simulink model "torqueBalancingPHRIStandup"  (Simulink 9.1)
settings: Solver=FixedStepDiscrete  StartTime=0.0  StopTime="Config.SIMULATION_TIME "  FixedStep=Config.Ts  RelTol=1e-3  EnableMultiTasking=on
StopFcn:
  | cd(fileparts(which(bdroot)));
  | stopTorqueBalancingPHRIStandup;
undefined symbols (not defined in the file or in its folder): ASSISTANT_DOF_FOR_SIMULINK, bVectorConstraintsFeet, bVectorConstraintsLegs, Config, ConstraintsMatrixFeet, ConstraintsMatrixLegs, Gain, Reg, ROBOT_DOF, ROBOT_DOF_FOR_SIMULINK, Sat, Sm
libraries: WBToolboxLibrary x154, simulink x4
(part 2 of 4)

== system torqueBalancingPHRIStandup/Robot system/Dynamics and Kinematics/Dynamics ==
  w_H_b : Inport
  qj : Inport  Port=2
  nu : Inport  Port=3
  Add motors reflected inertias : Subsystem
  Centroidal Momentum : WBToolboxLibrary/wholeBodyModel/Dynamics/Centroidal Momentum
      settings: SourceProductName=Whole Body Toolbox
  "CoM6D ->  CoMXYZ1" : Selector  InputPortWidth=6+ROBOT_DOF  IndexOptions=Index vector (dialog)  Indices=[7:6+ROBOT_DOF]  OutputSizes=1
  "CoM6D ->  CoMXYZ2" : Selector  InputPortWidth=6+ROBOT_DOF  IndexOptions=Index vector (dialog)  Indices=[1 2 3 4 5 6]  OutputSizes=1
  Get Bias Forces : WBToolboxLibrary/wholeBodyModel/Dynamics/Get Bias Forces
      settings: SourceProductName=Whole Body Toolbox
  Mass Matrix : WBToolboxLibrary/wholeBodyModel/Dynamics/Mass Matrix
      settings: SourceProductName=Whole Body Toolbox
  M(q) : Outport
  biasTorques : Outport  Port=2
  L(q,dq) : Outport  Port=3
  wires:
  Mass Matrix/1 -> Add motors reflected inertias/1(M)
  Centroidal Momentum/1 -> L(q,dq)/1
  Get Bias Forces/1 -> biasTorques/1
  w_H_b/1 -> Centroidal Momentum/1, Get Bias Forces/1, Mass Matrix/1
  qj/1 -> Centroidal Momentum/2, Get Bias Forces/2, Mass Matrix/2
  "CoM6D ->  CoMXYZ2"/1 -> Centroidal Momentum/3, Get Bias Forces/3
  "CoM6D ->  CoMXYZ1"/1 -> Centroidal Momentum/4, Get Bias Forces/4
  nu/1 -> "CoM6D ->  CoMXYZ1"/1, "CoM6D ->  CoMXYZ2"/1
  Add motors reflected inertias/1(M_with_motor_inertia) -> M(q)/1

== system torqueBalancingPHRIStandup/Robot system/Dynamics and Kinematics/Kinematics ==
  nu : Inport
  qj : Inport  Port=2
  w_H_b : Inport  Port=3
  "state " : Inport  Port=4
  Arm Contacts Kinematics : Subsystem
  "CoM6D ->  CoMXYZ3" : Selector  InputPortWidth=6+ROBOT_DOF  IndexOptions=Index vector (dialog)  Indices=[7:6+ROBOT_DOF]  OutputSizes=1
  "CoM6D ->  CoMXYZ4" : Selector  InputPortWidth=6+ROBOT_DOF  IndexOptions=Index vector (dialog)  Indices=[1 2 3 4 5 6]  OutputSizes=1
  Constant : Constant  Value=Config.iCubStandUp
  Contacts kinematics : Subsystem
  Jacobian com : WBToolboxLibrary/wholeBodyModel/Jacobians/Jacobian  frameName=Frames.COM
      settings: SourceProductName=Whole Body Toolbox
  Legs in Contact : MATLAB Function  TreatAsAtomicUnit=on
  xCom : Subsystem
  w_H_l_contact : Outport
  w_H_r_contact : Outport  Port=2
  J_l_contact : Outport  Port=3
  J_r_contact : Outport  Port=4
  J_CoM : Outport  Port=5
  xCoM : Outport  Port=6
  JDot_nu_l_contact : Outport  Port=7
  JDot_nu_r_contact : Outport  Port=8
  legsInContact : Outport  Port=9
  w_H_lArmContact : Outport  Port=10
  w_H_rArmContact : Outport  Port=11
  JLArm : Outport  Port=12
  JRArm : Outport  Port=13
  JDot_nu_lArm_contact : Outport  Port=14
  JDot_nu_rArm_contact : Outport  Port=15
  wires:
  nu/1 -> "CoM6D ->  CoMXYZ3"/1, "CoM6D ->  CoMXYZ4"/1
  w_H_b/1 -> Arm Contacts Kinematics/1(w_H_b1), Contacts kinematics/1(w_H_b), xCom/1(w_H_b), Jacobian com/1
  qj/1 -> Jacobian com/2, Arm Contacts Kinematics/2(qj1), Contacts kinematics/2(qj), xCom/2(qj)
  Jacobian com/1 -> J_CoM/1
  xCom/1(xCoM) -> xCoM/1
  "state "/1 -> Legs in Contact/2(state)
  Constant/1 -> Legs in Contact/1(icubStandup)
  "CoM6D ->  CoMXYZ3"/1 -> Arm Contacts Kinematics/4(dqj), Contacts kinematics/4(dqj)
  "CoM6D ->  CoMXYZ4"/1 -> Arm Contacts Kinematics/3(nu_b), Contacts kinematics/3(nu_b)
  Legs in Contact/1(legsInContact) -> Contacts kinematics/5(legsInContact), legsInContact/1
  Contacts kinematics/1(w_H_lContact) -> w_H_l_contact/1
  Contacts kinematics/2(w_H_rContact) -> w_H_r_contact/1
  Contacts kinematics/5(dJLnu) -> JDot_nu_l_contact/1
  Contacts kinematics/6(dJRnu) -> JDot_nu_r_contact/1
  Contacts kinematics/3(JL) -> J_l_contact/1
  Contacts kinematics/4(JR) -> J_r_contact/1
  Arm Contacts Kinematics/4(JRArm) -> JRArm/1
  Arm Contacts Kinematics/5(dJLArmnu) -> JDot_nu_lArm_contact/1
  Arm Contacts Kinematics/3(JLArm) -> JLArm/1
  Arm Contacts Kinematics/1(w_H_lArmContact) -> w_H_lArmContact/1
  Arm Contacts Kinematics/6(dJRArmnu) -> JDot_nu_rArm_contact/1
  Arm Contacts Kinematics/2(w_H_rArmContact) -> w_H_rArmContact/1

== system torqueBalancingPHRIStandup/Robot system/Robot State and References/Centroidal Momentum Matrix  ==
  w_H_b : Inport
  jointPos : Inport  Port=2
  CMM_LArm : Subsystem
  CMM_LLeg : Subsystem
  CMM_RArm : Subsystem
  CMM_RLeg : Subsystem
  CMM_base : Subsystem
  CMM_torso : Subsystem
  Matrix Concatenate6 : Concatenate  NumInputs=6  Mode=Multidimensional array  ConcatenateDimension=2
  CMM : Outport
  wires:
  Matrix Concatenate6/1 -> CMM/1
  CMM_base/1(CMM_base) -> Matrix Concatenate6/1
  CMM_torso/1(CMM_torso) -> Matrix Concatenate6/2
  CMM_LArm/1(CMM_LArm) -> Matrix Concatenate6/3
  jointPos/1 -> CMM_LArm/2(jointPos), CMM_RLeg/2(jointPos), CMM_LLeg/2(jointPos), CMM_RArm/2(jointPos), CMM_torso/2(jointPos), CMM_base/2(jointPos)
  w_H_b/1 -> CMM_LArm/1(w_H_b), CMM_RLeg/1(w_H_b), CMM_LLeg/1(w_H_b), CMM_RArm/1(w_H_b), CMM_torso/1(w_H_b), CMM_base/1(w_H_b)
  CMM_RArm/1(CMM_RArm) -> Matrix Concatenate6/4
  CMM_LLeg/1(CMM_LLeg) -> Matrix Concatenate6/5
  CMM_RLeg/1(CMM_RLeg) -> Matrix Concatenate6/6

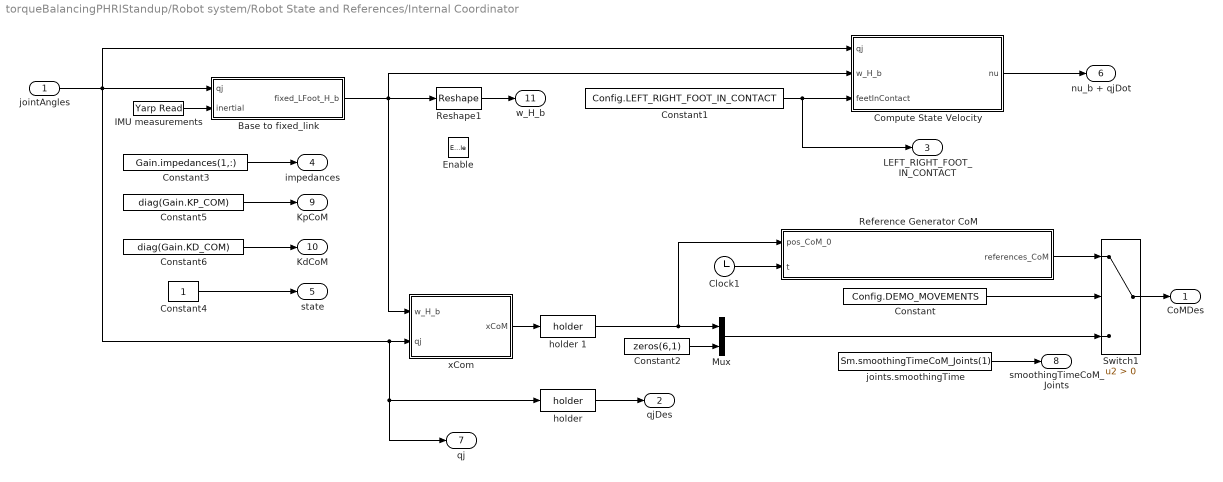
== system torqueBalancingPHRIStandup/Robot system/Robot State and References/Internal Coordinator ==
  jointAngles : Inport
  Enable : EnablePort
  Base to fixed_link : Subsystem
  Clock1 : Clock
  Compute State Velocity : Subsystem
  Constant : Constant  Value=Config.DEMO_MOVEMENTS
  Constant1 : Constant  Value=Config.LEFT_RIGHT_FOOT_IN_CONTACT
  Constant2 : Constant  Value=zeros(6,1)
  Constant3 : Constant  Value=Gain.impedances(1,:)
  Constant4 : Constant
  Constant5 : Constant  Value=diag(Gain.KP_COM)
  Constant6 : Constant  Value=diag(Gain.KD_COM)
  IMU measurements : WBToolboxLibrary/Utilities/Yarp Read  portName=Ports.IMU  signalSize=12  timeout=0.5  blocking=off  timestamp=off  autoconnect=on  errorOnConnection=on
      settings: SourceProductName=Whole Body Toolbox
  Mux : Mux  Inputs=2
  Reference Generator CoM : MATLAB Function  TreatAsAtomicUnit=on
  Reshape1 : Reshape  OutputDimensions=[4;4]
  Switch1 : Switch  Criteria=u2 > Threshold
  "holder " : WBToolboxLibrary/Utilities/holder 
      settings: SourceProductName=Whole Body Toolbox
  holder 1 : WBToolboxLibrary/Utilities/holder 
      settings: SourceProductName=Whole Body Toolbox
  joints.smoothingTime : Constant  Value=Sm.smoothingTimeCoM_Joints(1)
  xCom : Subsystem
  CoMDes : Outport
  qjDes : Outport  Port=2
  LEFT_RIGHT_FOOT_IN_CONTACT : Outport  Port=3
  impedances : Outport  Port=4
  state : Outport  Port=5
  nu_b + qjDot : Outport  Port=6
  qj : Outport  Port=7
  smoothingTimeCoM_Joints : Outport  Port=8
  KpCoM : Outport  Port=9
  KdCoM : Outport  Port=10
  w_H_b : Outport  Port=11
  wires:
  Constant/1 -> Switch1/2
  "holder "/1 -> qjDes/1
  Switch1/1 -> CoMDes/1
  Mux/1 -> Switch1/3
  Constant2/1 -> Mux/2
  Constant3/1 -> impedances/1
  Constant4/1 -> state/1
  Compute State Velocity/1(nu) -> nu_b + qjDot/1
  holder 1/1 -> Reference Generator CoM/1(pos_CoM_0), Mux/1
  Base to fixed_link/1(fixed_LFoot_H_b) -> Compute State Velocity/2(w_H_b), xCom/1(w_H_b), Reshape1/1
  xCom/1(xCoM) -> holder 1/1
  joints.smoothingTime/1 -> smoothingTimeCoM_Joints/1
  jointAngles/1 -> Compute State Velocity/1(qj), Base to fixed_link/1(qj), qj/1, "holder "/1, xCom/2(qj)
  Constant5/1 -> KpCoM/1
  Constant6/1 -> KdCoM/1
  Reshape1/1 -> w_H_b/1
  Constant1/1 -> Compute State Velocity/3("feetInContact "), LEFT_RIGHT_FOOT_IN_CONTACT/1
  IMU measurements/1 -> Base to fixed_link/2(inertial)
  Clock1/1 -> Reference Generator CoM/2(t)
  Reference Generator CoM/1(references_CoM) -> Switch1/1

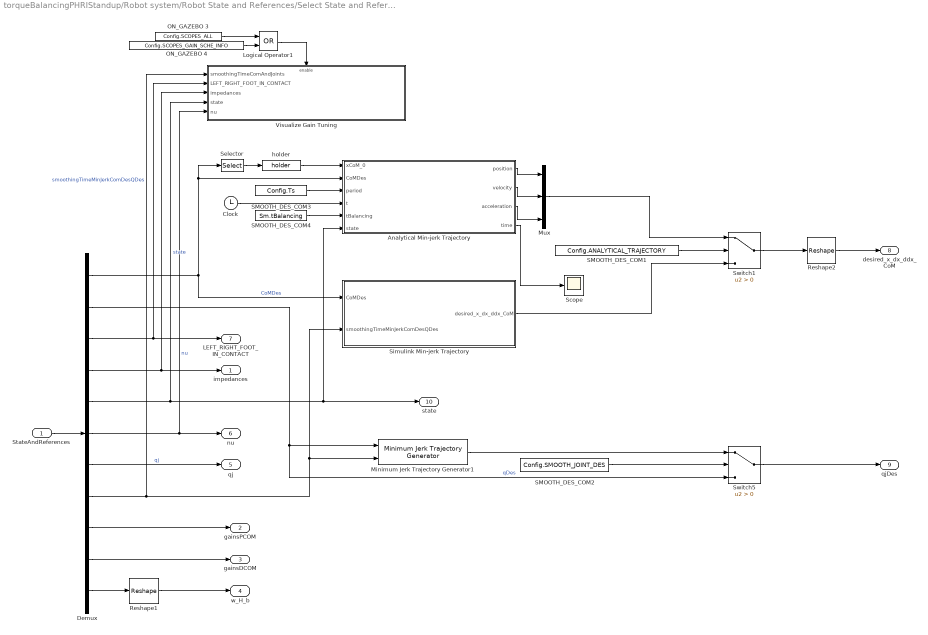
== system torqueBalancingPHRIStandup/Robot system/Robot State and References/Select State and References ==
  StateAndReferences : Inport
  Analytical Min-jerk Trajectory : MATLAB Function  TreatAsAtomicUnit=on
  Clock : Clock
  Demux : Demux  Outputs=[9,ROBOT_DOF,2,ROBOT_DOF,1,ROBOT_DOF+6,ROBOT_DOF,1,3,3,16]
  Logical Operator1 : Logic  Operator=OR  AllPortsSameDT=off  OutDataTypeStr=boolean
  Minimum Jerk Trajectory Generator1 : WBToolboxLibrary/Utilities/Minimum Jerk Trajectory Generator  externalSettlingTime=on  settlingTime=1  sampleTime=Config.Ts  resetOnSettlingTime=off  firstDerivatives=off  secondDerivatives=off  explicitInitialValue=off
      settings: SourceProductName=Whole Body Toolbox
  Mux : Mux  Inputs=3
  ON_GAZEBO 3 : Constant  Value=Config.SCOPES_ALL
  ON_GAZEBO 4 : Constant  Value=Config.SCOPES_GAIN_SCHE_INFO
  Reshape1 : Reshape  OutputDimensionality=Customize  OutputDimensions=[4;4]
  Reshape2 : Reshape  OutputDimensionality=Customize  OutputDimensions=[3,3]
  SMOOTH_DES_COM1 : Constant  Value=Config.ANALYTICAL_TRAJECTORY
  SMOOTH_DES_COM2 : Constant  Value=Config.SMOOTH_JOINT_DES
  SMOOTH_DES_COM3 : Constant  Value=Config.Ts
  SMOOTH_DES_COM4 : Constant  Value=Sm.tBalancing
  Scope : Scope
  Selector : Selector  InputPortWidth=9  IndexOptions=Index vector (dialog)  Indices=[1 2 3]  OutputSizes=1
  "Simulink Min-jerk Trajectory " : Subsystem
  Switch1 : Switch  Criteria=u2 > Threshold
  Switch5 : Switch  Criteria=u2 > Threshold
  "Visualize Gain Tuning  " : Subsystem
  "holder " : WBToolboxLibrary/Utilities/holder 
      settings: SourceProductName=Whole Body Toolbox
  impedances : Outport
  gainsPCOM : Outport  Port=2
  gainsDCOM : Outport  Port=3
  w_H_b : Outport  Port=4
  qj : Outport  Port=5
  nu : Outport  Port=6
  LEFT_RIGHT_FOOT_IN_CONTACT : Outport  Port=7
  desired_x_dx_ddx_CoM : Outport  Port=8
  qjDes : Outport  Port=9
  state : Outport  Port=10
  wires:
  SMOOTH_DES_COM2/1 -> Switch5/2
  Switch5/1 -> qjDes/1
  Demux/7 -> qj/1  "qj"
  Demux/11 -> Reshape1/1
  Demux/5 -> "Visualize Gain Tuning  "/4(state), Analytical Min-jerk Trajectory/6(state), state/1  "state"
  Demux/8 -> Minimum Jerk Trajectory Generator1/2, "Simulink Min-jerk Trajectory "/2(smoothingTimeMinJerkComDesQDes), "Visualize Gain Tuning  "/1(smoothingTimeComAndJoints)  "smoothingTimeMinJerkComDesQDes"
  Demux/2 -> Minimum Jerk Trajectory Generator1/1, Switch5/3  "qDes"
  Minimum Jerk Trajectory Generator1/1 -> Switch5/1
  Demux/6 -> "Visualize Gain Tuning  "/5(nu), nu/1  "nu"
  StateAndReferences/1 -> Demux/1
  Demux/4 -> "Visualize Gain Tuning  "/3(impedances), impedances/1
  Demux/3 -> "Visualize Gain Tuning  "/2(LEFT_RIGHT_FOOT_IN_CONTACT), LEFT_RIGHT_FOOT_IN_CONTACT/1
  Demux/9 -> gainsPCOM/1
  Demux/10 -> gainsDCOM/1
  Reshape1/1 -> w_H_b/1
  ON_GAZEBO 4/1 -> Logical Operator1/2
  ON_GAZEBO 3/1 -> Logical Operator1/1
  Logical Operator1/1 -> "Visualize Gain Tuning  "/Enable
  Demux/1 -> "Simulink Min-jerk Trajectory "/1(CoMDes), Selector/1, Analytical Min-jerk Trajectory/2(CoMDes)  "CoMDes"
  SMOOTH_DES_COM1/1 -> Switch1/2
  Switch1/1 -> Reshape2/1
  "Simulink Min-jerk Trajectory "/1(desired_x_dx_ddx_CoM) -> Switch1/3
  SMOOTH_DES_COM3/1 -> Analytical Min-jerk Trajectory/3(period)
  Clock/1 -> Analytical Min-jerk Trajectory/4(t)
  SMOOTH_DES_COM4/1 -> Analytical Min-jerk Trajectory/5(tBalancing)
  Reshape2/1 -> desired_x_dx_ddx_CoM/1
  Selector/1 -> "holder "/1
  "holder "/1 -> Analytical Min-jerk Trajectory/1(xCoM_0)
  Analytical Min-jerk Trajectory/1(position) -> Mux/1
  Analytical Min-jerk Trajectory/2(velocity) -> Mux/2
  Analytical Min-jerk Trajectory/3(acceleration) -> Mux/3
  Mux/1 -> Switch1/1
  Analytical Min-jerk Trajectory/4(time) -> Scope/1

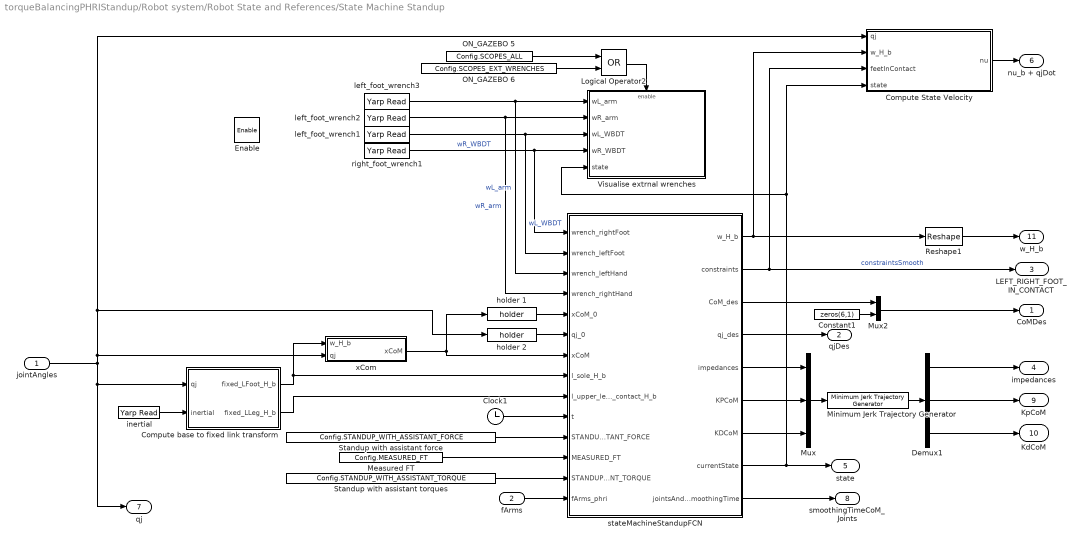
== system torqueBalancingPHRIStandup/Robot system/Robot State and References/State Machine Standup ==
  jointAngles : Inport
  fArms : Inport  Port=2
  Enable : EnablePort
  Clock1 : Clock
  Compute State Velocity : Subsystem
  Compute base to fixed link transform : Subsystem
  Constant1 : Constant  Value=zeros(6,1)
  Demux1 : Demux  Outputs=[ROBOT_DOF,3,3]
  Logical Operator2 : Logic  Operator=OR  AllPortsSameDT=off  OutDataTypeStr=boolean
  Measured FT : Constant  Value=Config.MEASURED_FT
  Minimum Jerk Trajectory Generator : WBToolboxLibrary/Utilities/Minimum Jerk Trajectory Generator  externalSettlingTime=off  settlingTime=Gain.SmoothingTimeGainScheduling  sampleTime=Config.Ts  resetOnSettlingTime=off  firstDerivatives=off  secondDerivatives=off  explicitInitialValue=off
      settings: SourceProductName=Whole Body Toolbox
  Mux : Mux  Inputs=3
  Mux2 : Mux  Inputs=2
  ON_GAZEBO 5 : Constant  Value=Config.SCOPES_ALL
  ON_GAZEBO 6 : Constant  Value=Config.SCOPES_EXT_WRENCHES
  Reshape1 : Reshape  OutputDimensions=[4;4]
  Standup with assistant force : Constant  Value=Config.STANDUP_WITH_ASSISTANT_FORCE
  Standup with assistant torques : Constant  Value=Config.STANDUP_WITH_ASSISTANT_TORQUE
  Visualise extrnal wrenches : Subsystem
  holder 1 : WBToolboxLibrary/Utilities/holder 
      settings: SourceProductName=Whole Body Toolbox
  holder 2 : WBToolboxLibrary/Utilities/holder 
      settings: SourceProductName=Whole Body Toolbox
  inertial : WBToolboxLibrary/Utilities/Yarp Read  portName=Ports.IMU  signalSize=12  timeout=0.5  blocking=off  timestamp=off  autoconnect=on  errorOnConnection=off
      settings: SourceProductName=Whole Body Toolbox
  left_foot_wrench1 : WBToolboxLibrary/Utilities/Yarp Read  portName=Ports.WBD_LEFTLEG_EE  signalSize=6  timeout=0.5  blocking=off  timestamp=off  autoconnect=on  errorOnConnection=on
      settings: SourceProductName=Whole Body Toolbox
  left_foot_wrench2 : WBToolboxLibrary/Utilities/Yarp Read  portName=Ports.RIGHT_ARM  signalSize=6  timeout=0.5  blocking=off  timestamp=off  autoconnect=on  errorOnConnection=on
      settings: SourceProductName=Whole Body Toolbox
  left_foot_wrench3 : WBToolboxLibrary/Utilities/Yarp Read  portName=Ports.LEFT_ARM  signalSize=6  timeout=0.5  blocking=off  timestamp=off  autoconnect=on  errorOnConnection=on
      settings: SourceProductName=Whole Body Toolbox
  right_foot_wrench1 : WBToolboxLibrary/Utilities/Yarp Read  portName=Ports.WBD_RIGHTLEG_EE  signalSize=6  timeout=0.5  blocking=off  timestamp=off  autoconnect=on  errorOnConnection=on
      settings: SourceProductName=Whole Body Toolbox
  stateMachineStandupFCN : MATLAB Function  TreatAsAtomicUnit=on
  xCom : Subsystem
  CoMDes : Outport
  qjDes : Outport  Port=2
  LEFT_RIGHT_FOOT_IN_CONTACT : Outport  Port=3
  impedances : Outport  Port=4
  state : Outport  Port=5
  nu_b + qjDot : Outport  Port=6
  qj : Outport  Port=7
  smoothingTimeCoM_Joints : Outport  Port=8
  KpCoM : Outport  Port=9
  KdCoM : Outport  Port=10
  w_H_b : Outport  Port=11
  wires:
  xCom/1(xCoM) -> holder 1/1, stateMachineStandupFCN/7(xCoM)
  stateMachineStandupFCN/4(qj_des) -> qjDes/1
  stateMachineStandupFCN/3(CoM_des) -> Mux2/1
  Mux2/1 -> CoMDes/1
  Constant1/1 -> Mux2/2
  stateMachineStandupFCN/8(currentState) -> Visualise extrnal wrenches/5(state), Compute State Velocity/4("state "), state/1
  stateMachineStandupFCN/2(constraints) -> Compute State Velocity/3("feetInContact "), LEFT_RIGHT_FOOT_IN_CONTACT/1  "constraintsSmooth"
  stateMachineStandupFCN/1(w_H_b) -> Compute State Velocity/2(w_H_b), Reshape1/1
  Compute State Velocity/1(nu) -> nu_b + qjDot/1
  stateMachineStandupFCN/9(jointsAndCoMSmoothingTime) -> smoothingTimeCoM_Joints/1
  stateMachineStandupFCN/6(KPCoM) -> Mux/2
  Demux1/3 -> KdCoM/1
  stateMachineStandupFCN/7(KDCoM) -> Mux/3
  stateMachineStandupFCN/5(impedances) -> Mux/1
  Mux/1 -> Minimum Jerk Trajectory Generator/1
  Minimum Jerk Trajectory Generator/1 -> Demux1/1
  Demux1/1 -> impedances/1
  Demux1/2 -> KpCoM/1
  jointAngles/1 -> Compute State Velocity/1(qj), holder 2/1, xCom/2(qj), qj/1, Compute base to fixed link transform/1(qj)
  Compute base to fixed link transform/1(fixed_LFoot_H_b) -> xCom/1(w_H_b), stateMachineStandupFCN/8(l_sole_H_b)
  Compute base to fixed link transform/2(fixed_LLeg_H_b) -> stateMachineStandupFCN/9(l_upper_leg_contact_H_b)
  inertial/1 -> Compute base to fixed link transform/2(inertial)
  Reshape1/1 -> w_H_b/1
  right_foot_wrench1/1 -> stateMachineStandupFCN/1(wrench_rightFoot), Visualise extrnal wrenches/4(wR_WBDT)  "wR_WBDT"
  left_foot_wrench1/1 -> stateMachineStandupFCN/2(wrench_leftFoot), Visualise extrnal wrenches/3(wL_WBDT)  "wL_WBDT"
  Logical Operator2/1 -> Visualise extrnal wrenches/Enable
  ON_GAZEBO 5/1 -> Logical Operator2/1
  ON_GAZEBO 6/1 -> Logical Operator2/2
  left_foot_wrench2/1 -> stateMachineStandupFCN/4(wrench_rightHand), Visualise extrnal wrenches/2(wR_arm)  "wR_arm"
  left_foot_wrench3/1 -> stateMachineStandupFCN/3(wrench_leftHand), Visualise extrnal wrenches/1(wL_arm)  "wL_arm"
  holder 1/1 -> stateMachineStandupFCN/5(xCoM_0)
  holder 2/1 -> stateMachineStandupFCN/6(qj_0)
  Clock1/1 -> stateMachineStandupFCN/10(t)
  Measured FT/1 -> stateMachineStandupFCN/12(MEASURED_FT)
  fArms/1 -> stateMachineStandupFCN/14(fArms_phri)
  Standup with assistant force/1 -> stateMachineStandupFCN/11(STANDUP_WITH_ASSISTANT_FORCE)
  Standup with assistant torques/1 -> stateMachineStandupFCN/13(STANDUP_WITH_ASSISTANT_TORQUE)

== system torqueBalancingPHRIStandup/Robot system/controller_QP/Compute angular momentum integral ==
  qjDes : Inport
  qj : Inport  Port=2
  constraints : Inport  Port=3
  state : Inport  Port=4
  Centroidal Momentum : WBToolboxLibrary/wholeBodyModel/Dynamics/Centroidal Momentum
      settings: SourceProductName=Whole Body Toolbox
  Compute base to fixed link transform : Subsystem
  Constant : Constant  Value=Config.iCubStandUp
  Fixed Links Jacobians : Subsystem
  Legs in Contact : MATLAB Function  TreatAsAtomicUnit=on
  References for H : MATLAB Function  TreatAsAtomicUnit=on
  Selector : Selector  InputPortWidth=6  IndexOptions=Index vector (dialog)  Indices=[4 5 6]  OutputSizes=1
  Sum : Sum  Inputs=|-+
  Switch : Switch  Criteria=u2 > Threshold  Threshold=0.1
  inertial : WBToolboxLibrary/Utilities/Yarp Read  portName=Ports.IMU  signalSize=12  timeout=0.5  blocking=off  timestamp=off  autoconnect=on  errorOnConnection=on
      settings: SourceProductName=Whole Body Toolbox
  intHw : Outport
  wires:
  qjDes/1 -> Sum/1, Compute base to fixed link transform/1(qj), Fixed Links Jacobians/2(qj), Centroidal Momentum/2
  qj/1 -> Sum/2
  Sum/1 -> Centroidal Momentum/4, References for H/1(qjErr)
  References for H/1(nu_b_equivalent) -> Centroidal Momentum/3
  Fixed Links Jacobians/1(J_LeftFixed) -> References for H/2(JL)
  Centroidal Momentum/1 -> Selector/1
  Selector/1 -> intHw/1
  Fixed Links Jacobians/2(J_RIghtFixed) -> References for H/3(JR)
  constraints/1 -> References for H/4(activeFeetConstraints)
  Switch/1 -> Centroidal Momentum/1, Fixed Links Jacobians/3(w_H_b)
  inertial/1 -> Compute base to fixed link transform/2(inertial)
  state/1 -> Legs in Contact/2(state)
  Constant/1 -> Legs in Contact/1(icubStandup)
  Legs in Contact/1(legsInContact) -> Fixed Links Jacobians/1("legsInContact "), Switch/2
  Compute base to fixed link transform/1(fixed_LLeg_H_b) -> Switch/1
  Compute base to fixed link transform/2(fixed_LFoot_H_b) -> Switch/3

== system torqueBalancingPHRIStandup/Robot system/controller_QP/Compute joint torques ==
  LEFT_RIGHT_FOOT_IN_CONTACT : Inport
  tauModel : Inport  Port=2
  Sigma : Inport  Port=3
  NA : Inport  Port=4
  fHDes : Inport  Port=5
  HessianMatrixQP1Foot : Inport  Port=6
  gradientQP1Foot : Inport  Port=7
  ConstraintsMatrixQP1Foot : Inport  Port=8
  bVectorConstraintsQP1Foot : Inport  Port=9
  HessianMatrixQP2Feet : Inport  Port=10
  gradientQP2Feet : Inport  Port=11
  ConstraintsMatrixQP2Feet : Inport  Port=12
  bVectorConstraintsQp2Feet : Inport  Port=13
  state : Inport  Port=14
  Add : Sum
  Add1 : Sum
  Product1 : Product  Multiplication=Matrix(*)
  Product2 : Product  Multiplication=Matrix(*)
  QPSolver : Subsystem
  Sum : Sum  Inputs=|++
  "tau " : Outport
  fDes QP : Outport  Port=2
  wires:
  NA/1 -> Product2/1
  QPSolver/1(f0OneFoot) -> Sum/2
  Product1/1 -> Add/2
  tauModel/1 -> Add/1
  Add/1 -> "tau "/1
  Add1/1 -> fDes QP/1, Product1/2
  Sum/1 -> Add1/1
  Product2/1 -> Add1/2
  Sigma/1 -> Product1/1
  QPSolver/2(f0TwoFeet) -> Product2/2
  gradientQP1Foot/1 -> QPSolver/3(gradientQP1Foot)
  ConstraintsMatrixQP2Feet/1 -> QPSolver/8(ConstraintsMatrixQP2Feet)
  LEFT_RIGHT_FOOT_IN_CONTACT/1 -> QPSolver/1(LEFT_RIGHT_FOOT_IN_CONTACT)
  bVectorConstraintsQP1Foot/1 -> QPSolver/5(bVectorConstraintsQP1Foot)
  HessianMatrixQP1Foot/1 -> QPSolver/2(HessianMatrixQP1Foot)
  ConstraintsMatrixQP1Foot/1 -> QPSolver/4(ConstraintsMatrixQP1Foot)
  gradientQP2Feet/1 -> QPSolver/7(gradientQP2Feet)
  HessianMatrixQP2Feet/1 -> QPSolver/6(HessianMatrixQP2Feet)
  bVectorConstraintsQp2Feet/1 -> QPSolver/9(bVectorConstraintsQp2Feet)
  state/1 -> QPSolver/10(state)
  fHDes/1 -> Sum/1

== system torqueBalancingPHRIStandup/Robot system/controller_QP/Compute joint torques (motor reflected inertia) ==
  u : Inport
  " " : Constant  Value=Config.USE_MOTOR_REFLECTED_INERTIA
  "(transpose(T*Gamma))^{-1}*I_m*(T*Gamma)^{-1}" : MATLAB Function  TreatAsAtomicUnit=on
  Add : Sum  Inputs=-+
  Gain : Gain  Gain=Config.K_ff
  Get Measurement : WBToolboxLibrary/wholeBodyStates/Get Measurement  measuredType=Joints Acceleration
      settings: SourceProductName=Whole Body Toolbox
  Product : Product  Multiplication=Matrix(*)
  Switch : Switch  Criteria=u2 > Threshold
  tau_joints : Outport
  wires:
  Get Measurement/1 -> Product/2
  Product/1 -> Gain/1
  Gain/1 -> Add/1
  Add/1 -> Switch/1
  " "/1 -> Switch/2
  Switch/1 -> tau_joints/1
  u/1 -> Add/2, Switch/3
  "(transpose(T*Gamma))^{-1}*I_m*(T*Gamma)^{-1}"/1(reflectedInertia) -> Product/1

== system torqueBalancingPHRIStandup/Robot system/controller_QP/Constraints ==
  legsInContact : Inport
  Constant : Constant  Value=ConstraintsMatrixFeet
  Constant1 : Constant  Value=bVectorConstraintsLegs
  Constant2 : Constant  Value=ConstraintsMatrixLegs
  Constant3 : Constant  Value=bVectorConstraintsFeet
  Switch1 : Switch  Criteria=u2 > Threshold  Threshold=0.1
  Switch2 : Switch  Criteria=u2 > Threshold  Threshold=0.1
  ConstraintsMatrix : Outport
  bVectorConstraints : Outport  Port=2
  wires:
  Constant2/1 -> Switch1/1
  Constant/1 -> Switch1/3
  Constant1/1 -> Switch2/1
  Constant3/1 -> Switch2/3
  legsInContact/1 -> Switch2/2, Switch1/2
  Switch1/1 -> ConstraintsMatrix/1
  Switch2/1 -> bVectorConstraints/1

== system torqueBalancingPHRIStandup/Robot system/synchronizer/GAZEBO_SYNCHRONIZER ==
  Enable : EnablePort
  Simulator Synchronizer : WBToolboxLibrary/Utilities/Simulator Synchronizer  period=Config.Ts  serverPortName='/clock/rpc'  clientPortName='/WBT_synchronizer/rpc:o'
      settings: SourceProductName=Whole Body Toolbox

== system torqueBalancingPHRIStandup/Robot system/synchronizer/REAL_TIME_SYNC ==
  Enable : EnablePort
  Real Time Synchronizer : WBToolboxLibrary/Utilities/Real Time Synchronizer  period=Config.Ts
      settings: SourceProductName=Whole Body Toolbox

== system torqueBalancingPHRIStandup/Assistant system/Real system/Contact Kinematics/Arm Contact Kinematics ==
  w_H_b : Inport
  qj : Inport  Port=2
  nu_b : Inport  Port=3
  qjdot : Inport  Port=4
  DotJ Nu : WBToolboxLibrary/wholeBodyModel/Jacobians/DotJ Nu  frameName=ASSISTANT_Frames.LEFT_HAND
      settings: SourceProductName=Whole Body Toolbox
  DotJ Nu1 : WBToolboxLibrary/wholeBodyModel/Jacobians/DotJ Nu  frameName=ASSISTANT_Frames.RIGHT_HAND
      settings: SourceProductName=Whole Body Toolbox
  Forward Kinematics : WBToolboxLibrary/wholeBodyModel/Kinematics/Forward Kinematics  frameName=ASSISTANT_Frames.LEFT_HAND
      settings: SourceProductName=Whole Body Toolbox
  Forward Kinematics1 : WBToolboxLibrary/wholeBodyModel/Kinematics/Forward Kinematics  frameName=ASSISTANT_Frames.RIGHT_HAND
      settings: SourceProductName=Whole Body Toolbox
  Jacobian : WBToolboxLibrary/wholeBodyModel/Jacobians/Jacobian  frameName=ASSISTANT_Frames.RIGHT_HAND
      settings: SourceProductName=Whole Body Toolbox
  Jacobian1 : WBToolboxLibrary/wholeBodyModel/Jacobians/Jacobian  frameName=ASSISTANT_Frames.LEFT_HAND
      settings: SourceProductName=Whole Body Toolbox
  w_H_lArm : Outport
  w_H_rArm : Outport  Port=2
  JLArm : Outport  Port=3
  JRArm : Outport  Port=4
  dJLArmnu : Outport  Port=5
  dJRArmnu : Outport  Port=6
  wires:
  Forward Kinematics/1 -> w_H_lArm/1
  Jacobian1/1 -> JLArm/1
  qjdot/1 -> DotJ Nu/4, DotJ Nu1/4
  w_H_b/1 -> Forward Kinematics/1, Jacobian/1, DotJ Nu1/1, DotJ Nu/1, Jacobian1/1, Forward Kinematics1/1
  qj/1 -> DotJ Nu1/2, DotJ Nu/2, Jacobian/2, Jacobian1/2, Forward Kinematics1/2, Forward Kinematics/2
  nu_b/1 -> DotJ Nu/3, DotJ Nu1/3
  Forward Kinematics1/1 -> w_H_rArm/1
  Jacobian/1 -> JRArm/1
  DotJ Nu1/1 -> dJRArmnu/1
  DotJ Nu/1 -> dJLArmnu/1

== system torqueBalancingPHRIStandup/Assistant system/Real system/Contact Kinematics/Leg Contact Kinematics ==
  w_H_b : Inport
  qj : Inport  Port=2
  nu_b : Inport  Port=3
  qjdot : Inport  Port=4
  DotJ Nu : WBToolboxLibrary/wholeBodyModel/Jacobians/DotJ Nu  frameName=ASSISTANT_Frames.LEFT_FOOT
      settings: SourceProductName=Whole Body Toolbox
  DotJ Nu1 : WBToolboxLibrary/wholeBodyModel/Jacobians/DotJ Nu  frameName=ASSISTANT_Frames.RIGHT_FOOT
      settings: SourceProductName=Whole Body Toolbox
  Forward Kinematics : WBToolboxLibrary/wholeBodyModel/Kinematics/Forward Kinematics  frameName=ASSISTANT_Frames.LEFT_FOOT
      settings: SourceProductName=Whole Body Toolbox
  Forward Kinematics1 : WBToolboxLibrary/wholeBodyModel/Kinematics/Forward Kinematics  frameName=ASSISTANT_Frames.RIGHT_FOOT
      settings: SourceProductName=Whole Body Toolbox
  Jacobian : WBToolboxLibrary/wholeBodyModel/Jacobians/Jacobian  frameName=ASSISTANT_Frames.RIGHT_FOOT
      settings: SourceProductName=Whole Body Toolbox
  Jacobian1 : WBToolboxLibrary/wholeBodyModel/Jacobians/Jacobian  frameName=ASSISTANT_Frames.LEFT_FOOT
      settings: SourceProductName=Whole Body Toolbox
  w_H_lFoot : Outport
  w_H_rFoot : Outport  Port=2
  JLFoot : Outport  Port=3
  JRFoot : Outport  Port=4
  dJLFootnu : Outport  Port=5
  dJRFootnu : Outport  Port=6
  wires:
  DotJ Nu/1 -> dJLFootnu/1
  DotJ Nu1/1 -> dJRFootnu/1
  Jacobian/1 -> JRFoot/1
  Forward Kinematics1/1 -> w_H_rFoot/1
  nu_b/1 -> DotJ Nu1/3, DotJ Nu/3
  qj/1 -> Forward Kinematics/2, Forward Kinematics1/2, Jacobian1/2, Jacobian/2, DotJ Nu/2, DotJ Nu1/2
  w_H_b/1 -> Forward Kinematics1/1, Jacobian1/1, DotJ Nu/1, DotJ Nu1/1, Jacobian/1, Forward Kinematics/1
  qjdot/1 -> DotJ Nu1/4, DotJ Nu/4
  Jacobian1/1 -> JLFoot/1
  Forward Kinematics/1 -> w_H_lFoot/1

== system torqueBalancingPHRIStandup/Assistant system/Real system/Dump and visualize/Assistant Data ==
  assistant_w_H_b : Inport
  assistant_jointData : Inport  Port=2
  assistant_jointVelocitiesData : Inport  Port=3
  assistant_jointTorquesData : Inport  Port=4
  Enable : EnablePort
  ON_GAZEBO 1 : Constant  Value=Config.USING_ROBOT_ASSISTANT
  ON_GAZEBO 3 : Constant  Value=Config.USING_HUMAN_ASSISTANT
  Selector : Selector  NumberOfDimensions=2  InputPortWidth=3  IndexOptions=Index vector (dialog),Index vector (dialog)  Indices=[1 2 3],[1 2 3]  OutputSizes=1,1
  Selector1 : Selector  NumberOfDimensions=2  InputPortWidth=3  IndexOptions=Index vector (dialog),Index vector (dialog)  Indices=[1 2 3],4  OutputSizes=1,1
  Using Human Assistant : Subsystem  Commented=on
  Using Robot Assistant : Subsystem
  base Pose : Scope  NumInputPorts=2
  wires:
  assistant_jointData/1 -> Using Human Assistant/1(assistant_jointData), Using Robot Assistant/1(assistant_jointData)
  assistant_jointVelocitiesData/1 -> Using Human Assistant/2(assistant_jointVelocitiesData), Using Robot Assistant/2(assistant_jointVelocitiesData)
  assistant_jointTorquesData/1 -> Using Human Assistant/3(assistant_jointTorquesData), Using Robot Assistant/3(assistant_jointTorquesData)
  Selector/1 -> base Pose/2  "baseOrientation"
  assistant_w_H_b/1 -> Selector1/1, Selector/1
  Selector1/1 -> base Pose/1  "basePosition"
  ON_GAZEBO 3/1 -> Using Human Assistant/Enable
  ON_GAZEBO 1/1 -> Using Robot Assistant/Enable

== system torqueBalancingPHRIStandup/Robot system/Dynamics and Kinematics/Dynamics/Add motors reflected inertias ==
  M : Inport
  Add motor reflected inertias : MATLAB Function  TreatAsAtomicUnit=on
  M_with_motor_inertia : Outport
  wires:
  M/1 -> Add motor reflected inertias/1(M)
  Add motor reflected inertias/1(M_with_inertia) -> M_with_motor_inertia/1

== system torqueBalancingPHRIStandup/Robot system/Dynamics and Kinematics/Kinematics/Arm Contacts Kinematics ==
  w_H_b1 : Inport
  qj1 : Inport  Port=2
  nu_b : Inport  Port=3
  dqj : Inport  Port=4
  " " : WBToolboxLibrary/wholeBodyModel/Jacobians/DotJ Nu  frameName=Frames.RIGHT_HAND
      settings: SourceProductName=Whole Body Toolbox
  "DotJ Nu l_sole " : WBToolboxLibrary/wholeBodyModel/Jacobians/DotJ Nu  frameName=Frames.LEFT_HAND
      settings: SourceProductName=Whole Body Toolbox
  Jacobian l_sole1 : WBToolboxLibrary/wholeBodyModel/Jacobians/Jacobian  frameName=Frames.LEFT_HAND
      settings: SourceProductName=Whole Body Toolbox
  Jacobian r_sole1 : WBToolboxLibrary/wholeBodyModel/Jacobians/Jacobian  frameName=Frames.RIGHT_HAND
      settings: SourceProductName=Whole Body Toolbox
  l_sole1 : WBToolboxLibrary/wholeBodyModel/Kinematics/Forward Kinematics  frameName=Frames.LEFT_HAND
      settings: SourceProductName=Whole Body Toolbox
  r_sole1 : WBToolboxLibrary/wholeBodyModel/Kinematics/Forward Kinematics  frameName=Frames.RIGHT_HAND
      settings: SourceProductName=Whole Body Toolbox
  w_H_lArmContact : Outport
  w_H_rArmContact : Outport  Port=2
  JLArm : Outport  Port=3
  JRArm : Outport  Port=4
  dJLArmnu : Outport  Port=5
  dJRArmnu : Outport  Port=6
  wires:
  w_H_b1/1 -> Jacobian l_sole1/1, " "/1, "DotJ Nu l_sole "/1, Jacobian r_sole1/1, r_sole1/1, l_sole1/1
  r_sole1/1 -> w_H_rArmContact/1
  dqj/1 -> "DotJ Nu l_sole "/4, " "/4
  nu_b/1 -> "DotJ Nu l_sole "/3, " "/3
  " "/1 -> dJRArmnu/1
  l_sole1/1 -> w_H_lArmContact/1
  Jacobian r_sole1/1 -> JRArm/1
  qj1/1 -> Jacobian l_sole1/2, " "/2, "DotJ Nu l_sole "/2, Jacobian r_sole1/2, r_sole1/2, l_sole1/2
  Jacobian l_sole1/1 -> JLArm/1
  "DotJ Nu l_sole "/1 -> dJLArmnu/1

== system torqueBalancingPHRIStandup/Robot system/Dynamics and Kinematics/Kinematics/Contacts kinematics ==
  w_H_b : Inport
  qj : Inport  Port=2
  nu_b : Inport  Port=3
  dqj : Inport  Port=4
  legsInContact : Inport  Port=5
  " " : WBToolboxLibrary/wholeBodyModel/Jacobians/DotJ Nu  frameName=Frames.RIGHT_LEG
      settings: SourceProductName=Whole Body Toolbox
  "    " : WBToolboxLibrary/wholeBodyModel/Jacobians/DotJ Nu  frameName=Frames.RIGHT_FOOT
      settings: SourceProductName=Whole Body Toolbox
  "DotJ Nu l_sole " : WBToolboxLibrary/wholeBodyModel/Jacobians/DotJ Nu  frameName=Frames.LEFT_FOOT
      settings: SourceProductName=Whole Body Toolbox
  DotJ Nu l_sole 1 : WBToolboxLibrary/wholeBodyModel/Jacobians/DotJ Nu  frameName=Frames.LEFT_LEG
      settings: SourceProductName=Whole Body Toolbox
  Jacobian l_sole : WBToolboxLibrary/wholeBodyModel/Jacobians/Jacobian  frameName=Frames.LEFT_FOOT
      settings: SourceProductName=Whole Body Toolbox
  Jacobian l_sole1 : WBToolboxLibrary/wholeBodyModel/Jacobians/Jacobian  frameName=Frames.LEFT_LEG
      settings: SourceProductName=Whole Body Toolbox
  Jacobian r_sole : WBToolboxLibrary/wholeBodyModel/Jacobians/Jacobian  frameName=Frames.RIGHT_FOOT
      settings: SourceProductName=Whole Body Toolbox
  Jacobian r_sole1 : WBToolboxLibrary/wholeBodyModel/Jacobians/Jacobian  frameName=Frames.RIGHT_LEG
      settings: SourceProductName=Whole Body Toolbox
  Switch{,1..5} (6 alike) : Switch  Criteria=u2 > Threshold  Threshold=0.1
  l_sole : WBToolboxLibrary/wholeBodyModel/Kinematics/Forward Kinematics  frameName=Frames.LEFT_FOOT
      settings: SourceProductName=Whole Body Toolbox
  l_sole1 : WBToolboxLibrary/wholeBodyModel/Kinematics/Forward Kinematics  frameName=Frames.LEFT_LEG
      settings: SourceProductName=Whole Body Toolbox
  r_sole : WBToolboxLibrary/wholeBodyModel/Kinematics/Forward Kinematics  frameName=Frames.RIGHT_FOOT
      settings: SourceProductName=Whole Body Toolbox
  r_sole1 : WBToolboxLibrary/wholeBodyModel/Kinematics/Forward Kinematics  frameName=Frames.RIGHT_LEG
      settings: SourceProductName=Whole Body Toolbox
  w_H_lContact : Outport
  w_H_rContact : Outport  Port=2
  JL : Outport  Port=3
  JR : Outport  Port=4
  dJLnu : Outport  Port=5
  dJRnu : Outport  Port=6
  wires:
  r_sole1/1 -> Switch/1
  r_sole/1 -> Switch/3
  l_sole1/1 -> Switch1/1
  l_sole/1 -> Switch1/3
  Switch1/1 -> w_H_lContact/1
  Switch/1 -> w_H_rContact/1
  w_H_b/1 -> Jacobian l_sole1/1, "DotJ Nu l_sole "/1, DotJ Nu l_sole 1/1, "    "/1, " "/1, Jacobian l_sole/1, Jacobian r_sole/1, Jacobian r_sole1/1, r_sole1/1, l_sole/1, l_sole1/1, r_sole/1
  Jacobian r_sole1/1 -> Switch2/1
  legsInContact/1 -> Switch1/2, Switch/2, Switch5/2, Switch4/2, Switch3/2, Switch2/2
  Jacobian r_sole/1 -> Switch2/3
  Jacobian l_sole1/1 -> Switch3/1
  Jacobian l_sole/1 -> Switch3/3
  Switch2/1 -> JR/1
  Switch3/1 -> JL/1
  qj/1 -> l_sole/2, "DotJ Nu l_sole "/2, DotJ Nu l_sole 1/2, "    "/2, " "/2, Jacobian l_sole/2, Jacobian l_sole1/2, Jacobian r_sole/2, Jacobian r_sole1/2, r_sole1/2, r_sole/2, l_sole1/2
  nu_b/1 -> "DotJ Nu l_sole "/3, DotJ Nu l_sole 1/3, "    "/3, " "/3
  dqj/1 -> "DotJ Nu l_sole "/4, DotJ Nu l_sole 1/4, " "/4, "    "/4
  " "/1 -> Switch4/1
  "    "/1 -> Switch4/3
  DotJ Nu l_sole 1/1 -> Switch5/1
  Switch4/1 -> dJRnu/1
  Switch5/1 -> dJLnu/1
  "DotJ Nu l_sole "/1 -> Switch5/3

== system torqueBalancingPHRIStandup/Robot system/Dynamics and Kinematics/Kinematics/xCom ==
  w_H_b : Inport
  qj : Inport  Port=2
  CoM : WBToolboxLibrary/wholeBodyModel/Kinematics/Forward Kinematics  frameName=Frames.COM
      settings: SourceProductName=Whole Body Toolbox
  "CoM6D ->  CoMXYZ2" : Selector  NumberOfDimensions=2  InputPortWidth=7  IndexOptions=Index vector (dialog),Index vector (dialog)  Indices=[1 2 3],[4]  OutputSizes=1,1
  xCoM : Outport
  wires:
  qj/1 -> CoM/2
  "CoM6D ->  CoMXYZ2"/1 -> xCoM/1
  CoM/1 -> "CoM6D ->  CoMXYZ2"/1
  w_H_b/1 -> CoM/1

== system torqueBalancingPHRIStandup/Robot system/Robot State and References/Centroidal Momentum Matrix /CMM_LArm ==
  w_H_b : Inport
  jointPos : Inport  Port=2
  Centroidal Momentum{1..2,19..20} (4 alike) : WBToolboxLibrary/wholeBodyModel/Dynamics/Centroidal Momentum
      settings: SourceProductName=Whole Body Toolbox
  Constant12 : Constant  Value=[0,0,0,1,0,0,0,0,0,0,0,0,0,0,0,0,0,0,0,0,0,0,0]
  Constant13 : Constant  Value=[0,0,0,0,1,0,0,0,0,0,0,0,0,0,0,0,0,0,0,0,0,0,0]
  Constant14 : Constant  Value=[0,0,0,0,0,1,0,0,0,0,0,0,0,0,0,0,0,0,0,0,0,0,0]
  Constant15 : Constant  Value=[0,0,0,0,0,0,1,0,0,0,0,0,0,0,0,0,0,0,0,0,0,0,0]
  Constant8 : Constant  Value=zeros(6,1)
  Matrix Concatenate2 : Concatenate  NumInputs=4  Mode=Multidimensional array  ConcatenateDimension=2
  CMM_LArm : Outport
  wires:
  Centroidal Momentum20/1 -> Matrix Concatenate2/2
  jointPos/1 -> Centroidal Momentum2/2, Centroidal Momentum1/2, Centroidal Momentum20/2, Centroidal Momentum19/2
  Constant13/1 -> Centroidal Momentum20/4
  Centroidal Momentum2/1 -> Matrix Concatenate2/4
  Centroidal Momentum19/1 -> Matrix Concatenate2/1
  Constant12/1 -> Centroidal Momentum19/4
  Centroidal Momentum1/1 -> Matrix Concatenate2/3
  Constant8/1 -> Centroidal Momentum2/3, Centroidal Momentum1/3, Centroidal Momentum20/3, Centroidal Momentum19/3
  Matrix Concatenate2/1 -> CMM_LArm/1
  Constant14/1 -> Centroidal Momentum1/4
  Constant15/1 -> Centroidal Momentum2/4
  w_H_b/1 -> Centroidal Momentum2/1, Centroidal Momentum1/1, Centroidal Momentum20/1, Centroidal Momentum19/1

== system torqueBalancingPHRIStandup/Robot system/Robot State and References/Centroidal Momentum Matrix /CMM_LLeg ==
  w_H_b : Inport
  jointPos : Inport  Port=2
  Centroidal Momentum{9..11,13..15} (6 alike) : WBToolboxLibrary/wholeBodyModel/Dynamics/Centroidal Momentum
      settings: SourceProductName=Whole Body Toolbox
  Constant21 : Constant  Value=[0,0,0,0,0,0,0,0,0,0,0,1,0,0,0,0,0,0,0,0,0,0,0]
  Constant22 : Constant  Value=[0,0,0,0,0,0,0,0,0,0,0,0,1,0,0,0,0,0,0,0,0,0,0]
  Constant23 : Constant  Value=[0,0,0,0,0,0,0,0,0,0,0,0,0,1,0,0,0,0,0,0,0,0,0]
  Constant25 : Constant  Value=zeros(6,1)
  Constant28 : Constant  Value=[0,0,0,0,0,0,0,0,0,0,0,0,0,0,1,0,0,0,0,0,0,0,0]
  Constant29 : Constant  Value=[0,0,0,0,0,0,0,0,0,0,0,0,0,0,0,1,0,0,0,0,0,0,0]
  Constant30 : Constant  Value=[0,0,0,0,0,0,0,0,0,0,0,0,0,0,0,0,1,0,0,0,0,0,0]
  Matrix Concatenate5 : Concatenate  NumInputs=6  Mode=Multidimensional array  ConcatenateDimension=2
  CMM_LLeg : Outport
  wires:
  Centroidal Momentum13/1 -> Matrix Concatenate5/4
  Centroidal Momentum9/1 -> Matrix Concatenate5/1
  Centroidal Momentum14/1 -> Matrix Concatenate5/5
  Centroidal Momentum15/1 -> Matrix Concatenate5/6
  Constant25/1 -> Centroidal Momentum15/3, Centroidal Momentum14/3, Centroidal Momentum13/3, Centroidal Momentum11/3, Centroidal Momentum10/3, Centroidal Momentum9/3
  Constant22/1 -> Centroidal Momentum10/4
  Centroidal Momentum10/1 -> Matrix Concatenate5/2
  Constant21/1 -> Centroidal Momentum9/4
  w_H_b/1 -> Centroidal Momentum15/1, Centroidal Momentum14/1, Centroidal Momentum13/1, Centroidal Momentum11/1, Centroidal Momentum10/1, Centroidal Momentum9/1
  jointPos/1 -> Centroidal Momentum15/2, Centroidal Momentum14/2, Centroidal Momentum13/2, Centroidal Momentum11/2, Centroidal Momentum10/2, Centroidal Momentum9/2
  Centroidal Momentum11/1 -> Matrix Concatenate5/3
  Matrix Concatenate5/1 -> CMM_LLeg/1
  Constant23/1 -> Centroidal Momentum11/4
  Constant28/1 -> Centroidal Momentum13/4
  Constant29/1 -> Centroidal Momentum14/4
  Constant30/1 -> Centroidal Momentum15/4

== system torqueBalancingPHRIStandup/Robot system/Robot State and References/Centroidal Momentum Matrix /CMM_RArm ==
  w_H_b : Inport
  jointPos : Inport  Port=2
  Centroidal Momentum{4..7} (4 alike) : WBToolboxLibrary/wholeBodyModel/Dynamics/Centroidal Momentum
      settings: SourceProductName=Whole Body Toolbox
  Constant17 : Constant  Value=[0,0,0,0,0,0,0,1,0,0,0,0,0,0,0,0,0,0,0,0,0,0,0]
  Constant18 : Constant  Value=[0,0,0,0,0,0,0,0,1,0,0,0,0,0,0,0,0,0,0,0,0,0,0]
  Constant19 : Constant  Value=[0,0,0,0,0,0,0,0,0,1,0,0,0,0,0,0,0,0,0,0,0,0,0]
  Constant20 : Constant  Value=[0,0,0,0,0,0,0,0,0,0,1,0,0,0,0,0,0,0,0,0,0,0,0]
  Constant24 : Constant  Value=zeros(6,1)
  Matrix Concatenate2 : Concatenate  NumInputs=4  Mode=Multidimensional array  ConcatenateDimension=2
  CMM_RArm : Outport
  wires:
  w_H_b/1 -> Centroidal Momentum7/1, Centroidal Momentum6/1, Centroidal Momentum5/1, Centroidal Momentum4/1
  Constant18/1 -> Centroidal Momentum5/4
  Constant17/1 -> Centroidal Momentum4/4
  jointPos/1 -> Centroidal Momentum7/2, Centroidal Momentum6/2, Centroidal Momentum5/2, Centroidal Momentum4/2
  Constant19/1 -> Centroidal Momentum6/4
  Constant20/1 -> Centroidal Momentum7/4
  Matrix Concatenate2/1 -> CMM_RArm/1
  Constant24/1 -> Centroidal Momentum7/3, Centroidal Momentum6/3, Centroidal Momentum5/3, Centroidal Momentum4/3
  Centroidal Momentum6/1 -> Matrix Concatenate2/3
  Centroidal Momentum5/1 -> Matrix Concatenate2/2
  Centroidal Momentum4/1 -> Matrix Concatenate2/1
  Centroidal Momentum7/1 -> Matrix Concatenate2/4

== system torqueBalancingPHRIStandup/Robot system/Robot State and References/Centroidal Momentum Matrix /CMM_RLeg ==
  w_H_b : Inport
  jointPos : Inport  Port=2
  Centroidal Momentum{12,26..30} (6 alike) : WBToolboxLibrary/wholeBodyModel/Dynamics/Centroidal Momentum
      settings: SourceProductName=Whole Body Toolbox
  Constant26 : Constant  Value=zeros(6,1)
  Constant31 : Constant  Value=[0,0,0,0,0,0,0,0,0,0,0,0,0,0,0,0,0,1,0,0,0,0,0]
  Constant32 : Constant  Value=[0,0,0,0,0,0,0,0,0,0,0,0,0,0,0,0,0,0,1,0,0,0,0]
  Constant33 : Constant  Value=[0,0,0,0,0,0,0,0,0,0,0,0,0,0,0,0,0,0,0,1,0,0,0]
  Constant34 : Constant  Value=[0,0,0,0,0,0,0,0,0,0,0,0,0,0,0,0,0,0,0,0,1,0,0]
  Constant35 : Constant  Value=[0,0,0,0,0,0,0,0,0,0,0,0,0,0,0,0,0,0,0,0,0,1,0]
  Constant36 : Constant  Value=[0,0,0,0,0,0,0,0,0,0,0,0,0,0,0,0,0,0,0,0,0,0,1]
  Matrix Concatenate4 : Concatenate  NumInputs=6  Mode=Multidimensional array  ConcatenateDimension=2
  CMM_RLeg : Outport
  wires:
  w_H_b/1 -> Centroidal Momentum12/1, Centroidal Momentum30/1, Centroidal Momentum29/1, Centroidal Momentum28/1, Centroidal Momentum27/1, Centroidal Momentum26/1
  jointPos/1 -> Centroidal Momentum12/2, Centroidal Momentum30/2, Centroidal Momentum29/2, Centroidal Momentum28/2, Centroidal Momentum27/2, Centroidal Momentum26/2
  Centroidal Momentum12/1 -> Matrix Concatenate4/6
  Centroidal Momentum29/1 -> Matrix Concatenate4/4
  Matrix Concatenate4/1 -> CMM_RLeg/1
  Centroidal Momentum28/1 -> Matrix Concatenate4/3
  Centroidal Momentum26/1 -> Matrix Concatenate4/1
  Centroidal Momentum27/1 -> Matrix Concatenate4/2
  Constant36/1 -> Centroidal Momentum12/4
  Constant31/1 -> Centroidal Momentum26/4
  Constant35/1 -> Centroidal Momentum30/4
  Constant32/1 -> Centroidal Momentum27/4
  Constant34/1 -> Centroidal Momentum29/4
  Constant26/1 -> Centroidal Momentum12/3, Centroidal Momentum30/3, Centroidal Momentum29/3, Centroidal Momentum28/3, Centroidal Momentum27/3, Centroidal Momentum26/3
  Constant33/1 -> Centroidal Momentum28/4
  Centroidal Momentum30/1 -> Matrix Concatenate4/5

== system torqueBalancingPHRIStandup/Robot system/Robot State and References/Centroidal Momentum Matrix /CMM_base ==
  w_H_b : Inport
  jointPos : Inport  Port=2
  Centroidal Momentum{21..25,31} (6 alike) : WBToolboxLibrary/wholeBodyModel/Dynamics/Centroidal Momentum
      settings: SourceProductName=Whole Body Toolbox
  Constant : Constant  Value=[1,0,0,0,0,0]
  Constant1 : Constant  Value=[0,1,0,0,0,0]
  Constant3 : Constant  Value=[0,0,0,1,0,0]
  Constant37 : Constant  Value=[0,0,1,0,0,0]
  Constant4 : Constant  Value=[0,0,0,0,1,0]
  Constant5 : Constant  Value=zeros(23,1)
  Constant6 : Constant  Value=[0,0,0,0,0,1]
  Matrix Concatenate : Concatenate  NumInputs=6  Mode=Multidimensional array  ConcatenateDimension=2
  CMM_base : Outport
  wires:
  w_H_b/1 -> Centroidal Momentum31/1, Centroidal Momentum25/1, Centroidal Momentum24/1, Centroidal Momentum23/1, Centroidal Momentum22/1, Centroidal Momentum21/1
  jointPos/1 -> Centroidal Momentum31/2, Centroidal Momentum25/2, Centroidal Momentum24/2, Centroidal Momentum23/2, Centroidal Momentum22/2, Centroidal Momentum21/2
  Centroidal Momentum25/1 -> Matrix Concatenate/5
  Matrix Concatenate/1 -> CMM_base/1
  Centroidal Momentum23/1 -> Matrix Concatenate/3
  Centroidal Momentum24/1 -> Matrix Concatenate/4
  Centroidal Momentum31/1 -> Matrix Concatenate/6
  Constant6/1 -> Centroidal Momentum31/3
  Constant/1 -> Centroidal Momentum21/3
  Constant1/1 -> Centroidal Momentum22/3
  Constant37/1 -> Centroidal Momentum23/3
  Constant5/1 -> Centroidal Momentum31/4, Centroidal Momentum25/4, Centroidal Momentum24/4, Centroidal Momentum23/4, Centroidal Momentum22/4, Centroidal Momentum21/4
  Constant4/1 -> Centroidal Momentum25/3
  Constant3/1 -> Centroidal Momentum24/3
  Centroidal Momentum22/1 -> Matrix Concatenate/2
  Centroidal Momentum21/1 -> Matrix Concatenate/1

== system torqueBalancingPHRIStandup/Robot system/Robot State and References/Centroidal Momentum Matrix /CMM_torso ==
  w_H_b : Inport
  jointPos : Inport  Port=2
  Centroidal Momentum16 : WBToolboxLibrary/wholeBodyModel/Dynamics/Centroidal Momentum
      settings: SourceProductName=Whole Body Toolbox
  Centroidal Momentum17 : WBToolboxLibrary/wholeBodyModel/Dynamics/Centroidal Momentum
      settings: SourceProductName=Whole Body Toolbox
  Centroidal Momentum18 : WBToolboxLibrary/wholeBodyModel/Dynamics/Centroidal Momentum
      settings: SourceProductName=Whole Body Toolbox
  Constant10 : Constant  Value=[0,1,0,0,0,0,0,0,0,0,0,0,0,0,0,0,0,0,0,0,0,0,0]
  Constant11 : Constant  Value=[0,0,1,0,0,0,0,0,0,0,0,0,0,0,0,0,0,0,0,0,0,0,0]
  Constant7 : Constant  Value=zeros(6,1)
  Constant9 : Constant  Value=[1,0,0,0,0,0,0,0,0,0,0,0,0,0,0,0,0,0,0,0,0,0,0]
  Matrix Concatenate1 : Concatenate  NumInputs=3  Mode=Multidimensional array  ConcatenateDimension=2
  CMM_torso : Outport
  wires:
  w_H_b/1 -> Centroidal Momentum18/1, Centroidal Momentum17/1, Centroidal Momentum16/1
  jointPos/1 -> Centroidal Momentum18/2, Centroidal Momentum17/2, Centroidal Momentum16/2
  Matrix Concatenate1/1 -> CMM_torso/1
  Centroidal Momentum18/1 -> Matrix Concatenate1/3
  Centroidal Momentum16/1 -> Matrix Concatenate1/1
  Constant10/1 -> Centroidal Momentum17/4
  Constant7/1 -> Centroidal Momentum18/3, Centroidal Momentum17/3, Centroidal Momentum16/3
  Constant11/1 -> Centroidal Momentum18/4
  Constant9/1 -> Centroidal Momentum16/4
  Centroidal Momentum17/1 -> Matrix Concatenate1/2

== system torqueBalancingPHRIStandup/Robot system/Robot State and References/Internal Coordinator/Base to fixed_link ==
  qj : Inport
  inertial : Inport  Port=2
  Constant1 : Constant  Value=Config.LEFT_FOOT_IN_CONTACT_AT_0
  Constant7 : Constant  Value=eye(4)
  "LFoot to base link transform " : Subsystem
  LFoot to world transform (fixed base) : WBToolboxLibrary/wholeBodyModel/Kinematics/Forward Kinematics  frameName=Frames.LEFT_FOOT
      settings: SourceProductName=Whole Body Toolbox
  RFoot to world transform (fixed base) : WBToolboxLibrary/wholeBodyModel/Kinematics/Forward Kinematics  frameName=Frames.RIGHT_FOOT
      settings: SourceProductName=Whole Body Toolbox
  Switch : Switch  Criteria=u2 > Threshold
  fixed_LFoot_H_b : Outport
  wires:
  "LFoot to base link transform "/1(link_H_b) -> fixed_LFoot_H_b/1
  inertial/1 -> "LFoot to base link transform "/2(inertial)
  qj/1 -> "LFoot to base link transform "/1(qj), RFoot to world transform (fixed base)/2, LFoot to world transform (fixed base)/2
  Constant7/1 -> LFoot to world transform (fixed base)/1, RFoot to world transform (fixed base)/1, "LFoot to base link transform "/4(w_H_base_fixed)
  Switch/1 -> "LFoot to base link transform "/3(w_H_link)
  LFoot to world transform (fixed base)/1 -> Switch/1
  RFoot to world transform (fixed base)/1 -> Switch/3
  Constant1/1 -> Switch/2

== system torqueBalancingPHRIStandup/Robot system/Robot State and References/Internal Coordinator/Compute State Velocity ==
  qj : Inport
  w_H_b : Inport  Port=2
  "feetInContact " : Inport  Port=3
  Compute Base Velocity : MATLAB Function  TreatAsAtomicUnit=on
  Feet Jacobians : Subsystem
  Get Measurement : WBToolboxLibrary/wholeBodyStates/Get Measurement  measuredType=Joints Velocity
      settings: SourceProductName=Whole Body Toolbox
  Mux : Mux  Inputs=2
  nu : Outport
  wires:
  Get Measurement/1 -> Mux/2, Compute Base Velocity/4(qjDot)
  Mux/1 -> nu/1
  "feetInContact "/1 -> Compute Base Velocity/3(feetInContact)
  Compute Base Velocity/1(nu_b) -> Mux/1
  qj/1 -> Feet Jacobians/1(qj)
  w_H_b/1 -> Feet Jacobians/2(w_H_b)
  Feet Jacobians/1(J_LFoot) -> Compute Base Velocity/1(J_LeftFoot)
  Feet Jacobians/2(J_RFoot) -> Compute Base Velocity/2(J_RightFoot)

== system torqueBalancingPHRIStandup/Robot system/Robot State and References/Internal Coordinator/xCom ==
  w_H_b : Inport
  qj : Inport  Port=2
  CoM : WBToolboxLibrary/wholeBodyModel/Kinematics/Forward Kinematics  frameName=Frames.COM
      settings: SourceProductName=Whole Body Toolbox
  "CoM6D ->  CoMXYZ2" : Selector  NumberOfDimensions=2  InputPortWidth=7  IndexOptions=Index vector (dialog),Index vector (dialog)  Indices=[1 2 3],[4]  OutputSizes=1,1
  xCoM : Outport
  wires:
  qj/1 -> CoM/2
  "CoM6D ->  CoMXYZ2"/1 -> xCoM/1
  CoM/1 -> "CoM6D ->  CoMXYZ2"/1
  w_H_b/1 -> CoM/1

== system torqueBalancingPHRIStandup/Robot system/Robot State and References/Select State and References/Simulink Min-jerk Trajectory  ==
  CoMDes : Inport
  smoothingTimeMinJerkComDesQDes : Inport  Port=2
  Minimum Jerk Trajectory Generator2 : WBToolboxLibrary/Utilities/Minimum Jerk Trajectory Generator  externalSettlingTime=on  settlingTime=0.1  sampleTime=Config.Ts  resetOnSettlingTime=off  firstDerivatives=on  secondDerivatives=on  explicitInitialValue=off
      settings: SourceProductName=Whole Body Toolbox
  Mux : Mux  Inputs=3
  Selector : Selector  InputPortWidth=9  IndexOptions=Index vector (dialog)  Indices=[1 2 3]  OutputSizes=1
  Switch1 : Switch  Criteria=u2 > Threshold
  Switch3 : Switch  Criteria=u2 > Threshold
  joints.smoothingTime : Constant  Value=Sm.smoothingTimeCoM
  desired_x_dx_ddx_CoM : Outport
  wires:
  Switch1/1 -> Minimum Jerk Trajectory Generator2/2
  Minimum Jerk Trajectory Generator2/2 -> Mux/2
  joints.smoothingTime/1 -> Switch1/3
  Mux/1 -> Switch3/1
  Switch3/1 -> desired_x_dx_ddx_CoM/1
  smoothingTimeMinJerkComDesQDes/1 -> Switch1/1, Switch1/2, Switch3/2
  Minimum Jerk Trajectory Generator2/3 -> Mux/3
  Selector/1 -> Minimum Jerk Trajectory Generator2/1
  Minimum Jerk Trajectory Generator2/1 -> Mux/1
  CoMDes/1 -> Switch3/3, Selector/1
